simulink model "SystemQ"  (R2014b)
settings: Solver=ode23  StartTime=0.0  StopTime=inf  RelTol=10e-3
PreLoadFcn:
  | initSysQ;
  | runSysQ;
undefined symbols (not defined in the file): Controllers, CR, dim, fdesignblkfcn, G, gcbh, lib, serial, Tjoint, Tpid, X, Y, Z
libraries: sm_lib x62, nesl_utility x28, simulink x10, roblocks x5, instrumentlib x2, dspmathops x1, dspinverses x1, dspmtrx3 x1
(part 1 of 3)
settings Model: Creator=Flavio  LastModifiedBy=Edoardo

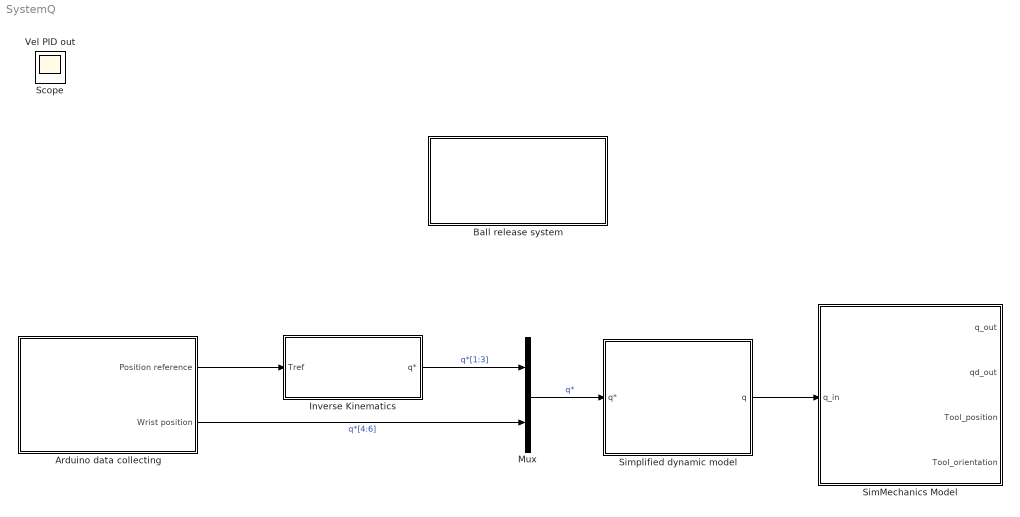
== system SystemQ ==
  Arduino data collecting : Subsystem
      mask Display:
      | image('Img/ardlogo.png',[0 0 0.75 1]);
      | port_label('output',1,'Pos. ref');
      | port_label('output',2,'Wrist joints');
  Ball release system : Subsystem
  Inverse Kinematics : Subsystem  mask{Jd=0.05, K=5}
      mask prompts: Jd "Jacobian damping"; K "Error gain"
  Mux : Mux  Inputs=2
  SimMechanics Model : Subsystem
      mask Display:
      | image('Img/simmech.png',[0.1 0.1 0.8 0.8]);
      | port_label('input',1,'q_in');
  Simplified dynamic model : Subsystem
      mask Display:
      | image('Img/dcmotor.jpg',[0.1 0.1 0.8 0.8]);
      | port_label('input',1,'q*');
      | port_label('output',1,'q');
  Scope : Scope
      settings: YMin=0  YMax=7  SaveName=ScopeData4
  Vel PID out : Scope
      settings: ShowLegends=on  YMin=-15  YMax=15  Decimation=10
  wires:
  Simplified dynamic model/1(q) -> SimMechanics Model/1("q_in ")
  Arduino data collecting/1(Position reference) -> Inverse Kinematics/1(Tref)
  Arduino data collecting/2(Wrist position) -> Mux/2  "q*[4:6]"
  Inverse Kinematics/1(q*) -> Mux/1  "q*[1:3]"
  Mux/1 -> Simplified dynamic model/1(q*)  "q*"

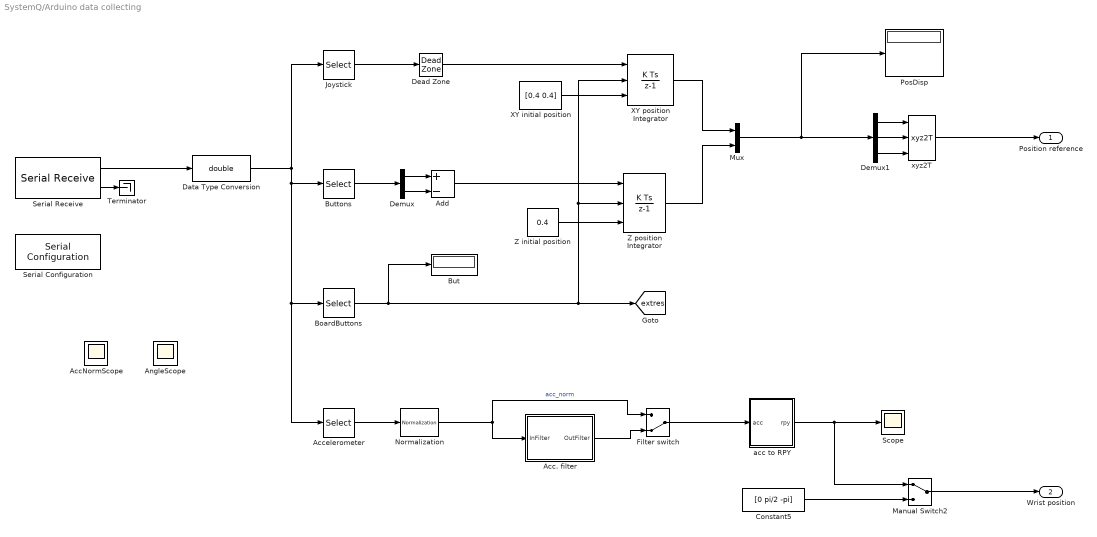
== system SystemQ/Arduino data collecting ==
  Acc. filter : Subsystem
  AccNormScope : Scope
      settings: Floating=on  ShowLegends=on  YMin=0  YMax=1  SaveName=ScopeData3
  Accelerometer : Selector  InputPortWidth=8  Indices=[5 6 7]
  Add : Sum  Inputs=+-
  AngleScope : Scope
      settings: Floating=on  ShowLegends=on  YMin=-0.2  YMax=1.6
  BoardButtons : Selector  InputPortWidth=8  Indices=8
  But : Display
  Buttons : Selector  InputPortWidth=8  Indices=[3 4]
  Constant5 : Constant  Value=[0 pi/2 -pi]
  Data Type Conversion : DataTypeConversion  OutDataTypeStr=double
  Dead Zone : DeadZone  LowerValue=-20  UpperValue=20  SaturateOnIntegerOverflow=on
  Demux : Demux  Outputs=2
  Demux1 : Demux  Outputs=3
  Filter switch : ManualSwitch  CurrentSetting=0
  Joystick : Selector  InputPortWidth=8  Indices=[1 2]
  Manual Switch2 : ManualSwitch
  Mux : Mux  Inputs=2
  Normalization : dspmathops/Normalization  NormType=2-norm  Bias=1e-10  NormOver=Each column  ColComp=on  Dimension=1  outputDataTypeStr=Inherit: Same as product output  outputLastDataTypeStr=Inherit: Same as product output  outputMin=[]  outputMax=[]  accumDataTypeStr=Inherit: Same as product output  accumLastDataTypeStr=Inherit: Same as product output  roundingMode=Floor  overflowMode=off
  PosDisp : Display
  Scope : Scope
      settings: SaveName=ScopeData2
  Serial Configuration : instrumentlib/Serial Configuration  Priority=-200000  ComPortMenu=<Please select a port...>  ComPort=COM5  ObjConstructor=serial('COM5');  BaudRate=115200  DataBits=8  Parity=none  StopBits=1  FlowControl=none  Timeout=10  ByteOrder=LittleEndian
  Serial Receive : instrumentlib/Serial Receive  ComPortMenu=<Please select a port...>  ComPort=COM5  ObjConstructor=serial('COM5');  Header=\a  Terminator=CR ('\r')  DataSize=8  DataType=int16  EnableBlockingMode=off  ActionDataUnavailable=Output last received value  CustomValue=0  SampleTime=0.1
  Terminator : Terminator
  XY initial position : Constant  Value=[0.4 0.4]
  XY position Integrator : DiscreteIntegrator  gainval=0.0001  ExternalReset=falling  InitialConditionSource=external  InitialCondition=[0.6181 0.4]  InitialConditionSetting=State (most efficient)  SampleTime=-1  UpperSaturationLimit=0.5  LowerSaturationLimit=-0.5
  Z initial position : Constant  Value=0.4
  Z position Integrator : DiscreteIntegrator  gainval=0.01  ExternalReset=falling  InitialConditionSource=external  InitialCondition=0.0875  InitialConditionSetting=State (most efficient)  SampleTime=-1  UpperSaturationLimit=0.6  LowerSaturationLimit=-0.6
  acc to RPY : Subsystem
  xyz2T : roblocks/Transform Conversion/xyz2T
  Position reference : Outport
  Wrist position : Outport  Port=2
  tag scope: extres=global
  wires:
  Demux1/1 -> xyz2T/1
  Add/1 -> Z position Integrator/1
  XY position Integrator/1 -> Mux/1
  Normalization/1 -> Filter switch/1, Acc. filter/1(InFilter)  "acc_norm"
  Data Type Conversion/1 -> BoardButtons/1, Accelerometer/1, Buttons/1, Joystick/1
  XY initial position/1 -> XY position Integrator/3
  Demux1/2 -> xyz2T/2
  Buttons/1 -> Demux/1
  Z position Integrator/1 -> Mux/2
  Joystick/1 -> Dead Zone/1
  Demux1/3 -> xyz2T/3
  Z initial position/1 -> Z position Integrator/3
  Mux/1 -> Demux1/1, PosDisp/1
  Dead Zone/1 -> XY position Integrator/1
  Filter switch/1 -> acc to RPY/1(acc)
  Acc. filter/1(OutFilter) -> Filter switch/2
  Demux/2 -> Add/2
  Demux/1 -> Add/1
  Accelerometer/1 -> Normalization/1
  Serial Receive/1 -> Data Type Conversion/1
  Serial Receive/2 -> Terminator/1
  xyz2T/1 -> Position reference/1
  Manual Switch2/1 -> Wrist position/1
  acc to RPY/1(rpy) -> Scope/1, Manual Switch2/1
  Constant5/1 -> Manual Switch2/2
  BoardButtons/1 -> But/1, XY position Integrator/2, Z position Integrator/2, [extres]

== system SystemQ/Ball release system ==
  BallChart : Stateflow chart  TreatAsAtomicUnit=on
  Memory error x : Memory  X0=1
  Memory error x1 : Memory  X0=1
  tag scope: Status=global
  wires:
  Memory error x/1 -> BallChart/1(error1)
  [ER1] -> Memory error x/1
  [ER2] -> Memory error x1/1
  Memory error x1/1 -> BallChart/2(error2)
  BallChart/1(status) -> [Status]

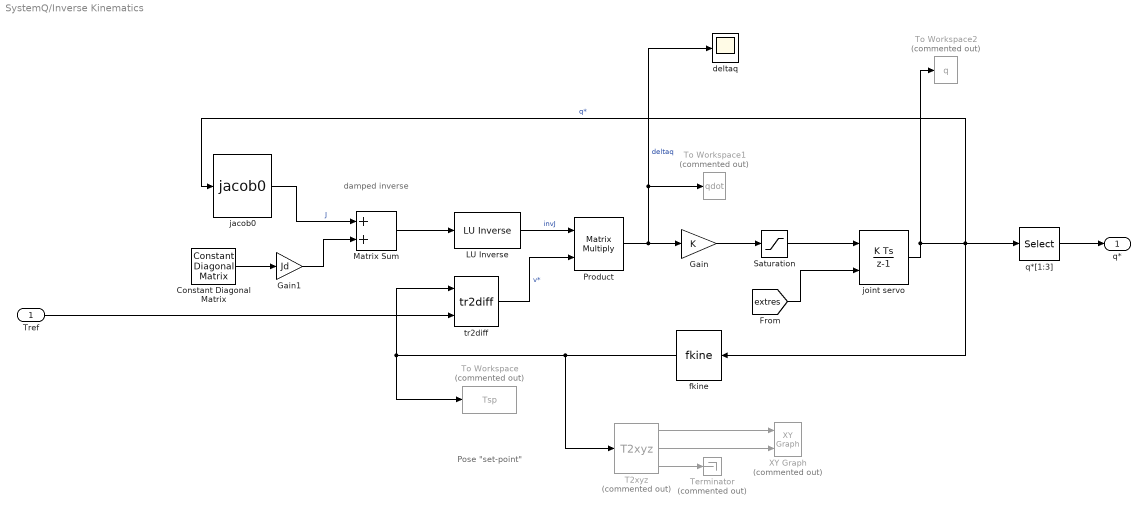
== system SystemQ/Inverse Kinematics ==
  note: Pose "set-point"
  note: damped inverse
  Tref : Inport
  " LU Inverse" : dspinverses/ LU Inverse
  Constant Diagonal Matrix : dspmtrx3/Constant Diagonal Matrix  q=ones(1,6)  frame=off  dataType=Inherit from 'Constant(s) along diagonal'  isSigned=on  wordLen=16  udDataType=sfix(16)  fracBitsMode=Best precision  numFracBits=15
  Gain : Gain  Gain=K  SaturateOnIntegerOverflow=on  OutDataTypeStr=Inherit: Same as input  ParamDataTypeStr=Inherit: Same as input
  Gain1 : Gain  Gain=Jd
  Matrix Sum : Sum
  Product : Product  Multiplication=Matrix(*)  SaturateOnIntegerOverflow=on  RndMeth=Zero  InputSameDT=on  OutDataTypeStr=Inherit: Same as first input
  Saturation : Saturate  UpperLimit=10  LowerLimit=-10
  T2xyz : roblocks/Transform Conversion/T2xyz  Commented=on
  Terminator : Terminator  Commented=on
  To Workspace : ToWorkspace  Commented=on  VariableName=Tsp  SampleTime=-1
  To Workspace1 : ToWorkspace  Commented=on  VariableName=qdot  SampleTime=-1
  To Workspace2 : ToWorkspace  Commented=on  VariableName=q  SampleTime=-1
  XY Graph : simulink/Sinks/XY Graph  Commented=on  xmin=-1  xmax=1  ymin=-1  ymax=1  st=-1
  deltaq : Scope
      settings: YMin=-2.5e-13  YMax=2.5e-13  SaveName=ScopeData7
  fkine : roblocks/Kinematics/fkine  robot=robot
  "jacob0 " : roblocks/Kinematics/jacob0   robot=robot
  joint servo : DiscreteIntegrator  ExternalReset=falling  InitialCondition=qn'  SampleTime=Tjoint  UpperSaturationLimit=pi  LowerSaturationLimit=-pi
  q*[1:3] : Selector  InputPortWidth=6  Indices=[1 2 3]
  tr2diff : roblocks/Kinematics/tr2diff  robot=robot
  q* : Outport
  wires:
  Constant Diagonal Matrix/1 -> Gain1/1
  Gain/1 -> Saturation/1
  " LU Inverse"/1 -> Product/1  "invJ"
  fkine/1 -> T2xyz/1, To Workspace/1, tr2diff/1
  Tref/1 -> tr2diff/2
  T2xyz/1 -> XY Graph/1
  Gain1/1 -> Matrix Sum/2
  "jacob0 "/1 -> Matrix Sum/1  "J"
  tr2diff/1 -> Product/2  "v*"
  T2xyz/2 -> XY Graph/2
  Matrix Sum/1 -> " LU Inverse"/1
  Product/1 -> deltaq/1, To Workspace1/1, Gain/1  "deltaq"
  T2xyz/3 -> Terminator/1
  joint servo/1 -> To Workspace2/1, fkine/1, "jacob0 "/1, q*[1:3]/1  "q*"
  [extres] -> joint servo/2
  Saturation/1 -> joint servo/1
  q*[1:3]/1 -> q*/1

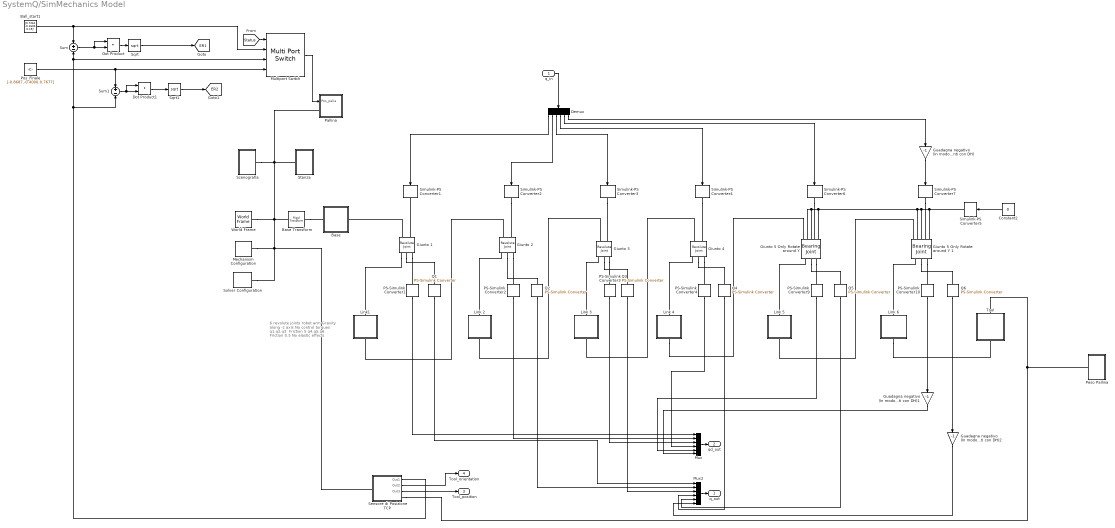
== system SystemQ/SimMechanics Model ==
  note: 6 revolute joints robot arm
      | Gravity along -z axis
      | No control torques
      | q1,q2,q3: Friction 5
      |  q4,q5,q6: Friction 0.5
      | No elastic effects
  "q_in " : Inport
  Ball_start1 : Constant  Value=[0.7261 -0.1604 0.15]'
  Base : Subsystem  mask(Double Pendulum Base){R=20, B_T=5, C_L=65, rp=5, clr=[0.5 0.5 0.5], Ro=dim.ro}
      mask prompts: R "Base radius (cm):"; B_T "Base thickeness (cm):"; C_L "Lunghezza cilindro (cm)"; rp "Peg radius (cm):"; clr "Base color:"; Ro "Densità (Kg/m^3):"
      mask help: Base body of the double pendulum mechanism.
  Base Transform : sm_lib/Frames and Transforms/Rigid Transform  TranslationMethod=None  TranslationLengthUnit=m  TranslationStandardAxis=+Z  TranslationStandardOffset=0  TranslationCartesianOffset=[0 0 0]  TranslationROffset=0  TranslationROffsetUnits=m  TranslationZOffset=0  TranslationZOffsetUnits=m  TranslationThetaOffset=0  TranslationThetaOffsetUnits=deg  RotationMethod=None  RotationAngleUnits=deg  RotationStandardAxis=+Z  RotationAngle=0  RotationArbitraryAxis=[0 0 1]  FollAlignAxisA=+Z  BaseAlignAxisA=-Y  FollAlignAxisB=+Y  BaseAlignAxisB=+X  RotationMatrix=[1 0 0; 0 1 0; 0 0 1]  BlockFunction=simmechanics.library.frames_transforms.rigid_transform
  Constant2 : Constant  Value=0
  Demux : Demux  Outputs=6
  Dot Product : DotProduct  InputSameDT=on  OutDataTypeStr=Inherit: Inherit via internal rule
  Dot Product1 : DotProduct  InputSameDT=on  OutDataTypeStr=Inherit: Inherit via internal rule
  Giunto 1 : sm_lib/Joints/Revolute Joint  SenseConstraintForce=off  SenseConstraintForceX=off  SenseConstraintForceY=off  SenseConstraintForceZ=off  SenseConstraintTorque=off  SenseConstraintTorqueX=off  SenseConstraintTorqueY=off  SenseConstraintTorqueZ=off  SenseTotalForce=off  SenseTotalForceX=off  SenseTotalForceY=off  SenseTotalForceZ=off  SenseTotalTorque=off  SenseTotalTorqueX=off  SenseTotalTorqueY=off  SenseTotalTorqueZ=off  CompositeWrenchDir=FollowerOnBase  CompositeWrenchFrame=BaseFrame  EquilibriumPosition=0  EquilibriumPositionUnits=rad  SpringStiffness=0  SpringStiffnessUnits=N*m/rad  DampingCoefficient=5  DampingCoefficientUnits=N*m/(rad/s)  TorqueActuationMode=ComputedTorque  MotionActuationMode=InputMotion  SensePosition=on  SenseVelocity=on  SenseAcceleration=off  SenseTorqueForce=off  PositionTargetValue=0  PositionTargetValueUnits=rad  PositionTargetSpecify=on  PositionTargetPriority=High  VelocityTargetValue=0  VelocityTargetValueUnits=rad/s  VelocityTargetSpecify=off  VelocityTargetPriority=Low  BlockFunction=simmechanics.library.joints.revolute_joint
  Giunto 2 : sm_lib/Joints/Revolute Joint  SenseConstraintForce=off  SenseConstraintForceX=off  SenseConstraintForceY=off  SenseConstraintForceZ=off  SenseConstraintTorque=off  SenseConstraintTorqueX=off  SenseConstraintTorqueY=off  SenseConstraintTorqueZ=off  SenseTotalForce=off  SenseTotalForceX=off  SenseTotalForceY=off  SenseTotalForceZ=off  SenseTotalTorque=off  SenseTotalTorqueX=off  SenseTotalTorqueY=off  SenseTotalTorqueZ=off  CompositeWrenchDir=FollowerOnBase  CompositeWrenchFrame=BaseFrame  EquilibriumPosition=0  EquilibriumPositionUnits=rad  SpringStiffness=0  SpringStiffnessUnits=N*m/rad  DampingCoefficient=5  DampingCoefficientUnits=N*m/(rad/s)  TorqueActuationMode=ComputedTorque  MotionActuationMode=InputMotion  SensePosition=on  SenseVelocity=on  SenseAcceleration=off  SenseTorqueForce=off  PositionTargetValue=pi/2  PositionTargetValueUnits=rad  PositionTargetSpecify=on  PositionTargetPriority=High  VelocityTargetValue=0  VelocityTargetValueUnits=rad/s  VelocityTargetSpecify=off  VelocityTargetPriority=Low  BlockFunction=simmechanics.library.joints.revolute_joint
  Giunto 3 : sm_lib/Joints/Revolute Joint  SenseConstraintForce=off  SenseConstraintForceX=off  SenseConstraintForceY=off  SenseConstraintForceZ=off  SenseConstraintTorque=off  SenseConstraintTorqueX=off  SenseConstraintTorqueY=off  SenseConstraintTorqueZ=off  SenseTotalForce=off  SenseTotalForceX=off  SenseTotalForceY=off  SenseTotalForceZ=off  SenseTotalTorque=off  SenseTotalTorqueX=off  SenseTotalTorqueY=off  SenseTotalTorqueZ=off  CompositeWrenchDir=FollowerOnBase  CompositeWrenchFrame=BaseFrame  EquilibriumPosition=pi/4  EquilibriumPositionUnits=rad  SpringStiffness=0  SpringStiffnessUnits=N*m/rad  DampingCoefficient=5  DampingCoefficientUnits=N*m/(rad/s)  TorqueActuationMode=ComputedTorque  MotionActuationMode=InputMotion  SensePosition=on  SenseVelocity=on  SenseAcceleration=off  SenseTorqueForce=off  PositionTargetValue=-(pi*5/6)  PositionTargetValueUnits=rad  PositionTargetSpecify=on  PositionTargetPriority=High  VelocityTargetValue=0  VelocityTargetValueUnits=rad/s  VelocityTargetSpecify=off  VelocityTargetPriority=Low  BlockFunction=simmechanics.library.joints.revolute_joint
  Giunto 4 : sm_lib/Joints/Revolute Joint  SenseConstraintForce=off  SenseConstraintForceX=off  SenseConstraintForceY=off  SenseConstraintForceZ=off  SenseConstraintTorque=off  SenseConstraintTorqueX=off  SenseConstraintTorqueY=off  SenseConstraintTorqueZ=off  SenseTotalForce=off  SenseTotalForceX=off  SenseTotalForceY=off  SenseTotalForceZ=off  SenseTotalTorque=off  SenseTotalTorqueX=off  SenseTotalTorqueY=off  SenseTotalTorqueZ=off  CompositeWrenchDir=FollowerOnBase  CompositeWrenchFrame=BaseFrame  EquilibriumPosition=0  EquilibriumPositionUnits=rad  SpringStiffness=0  SpringStiffnessUnits=N*m/rad  DampingCoefficient=0.5  DampingCoefficientUnits=N*m/(rad/s)  TorqueActuationMode=ComputedTorque  MotionActuationMode=InputMotion  SensePosition=on  SenseVelocity=on  SenseAcceleration=off  SenseTorqueForce=off  PositionTargetValue=0  PositionTargetValueUnits=rad  PositionTargetSpecify=on  PositionTargetPriority=High  VelocityTargetValue=0  VelocityTargetValueUnits=rad/s  VelocityTargetSpecify=off  VelocityTargetPriority=Low  BlockFunction=simmechanics.library.joints.revolute_joint
  "Giunto 5 Only Rotate around Y " : sm_lib/Joints/Bearing Joint  SenseConstraintForce=off  SenseConstraintForceX=off  SenseConstraintForceY=off  SenseConstraintForceZ=off  SenseConstraintTorque=off  SenseConstraintTorqueX=off  SenseConstraintTorqueY=off  SenseConstraintTorqueZ=off  SenseTotalForce=off  SenseTotalForceX=off  SenseTotalForceY=off  SenseTotalForceZ=off  SenseTotalTorque=off  SenseTotalTorqueX=off  SenseTotalTorqueY=off  SenseTotalTorqueZ=off  CompositeWrenchDir=FollowerOnBase  CompositeWrenchFrame=BaseFrame  PzEquilibriumPosition=0  PzEquilibriumPositionUnits=m  PzSpringStiffness=0  PzSpringStiffnessUnits=N/m  PzDampingCoefficient=0  PzDampingCoefficientUnits=N/(m/s)  PzTorqueActuationMode=ComputedTorque  PzMotionActuationMode=InputMotion  PzSensePosition=off  PzSenseVelocity=off  PzSenseAcceleration=off  PzSenseTorqueForce=off  PzPositionTargetValue=0  PzPositionTargetValueUnits=m  PzPositionTargetSpecify=on  PzPositionTargetPriority=High  PzVelocityTargetValue=0  PzVelocityTargetValueUnits=m/s  PzVelocityTargetSpecify=off  PzVelocityTargetPriority=High  RxEquilibriumPosition=0  RxEquilibriumPositionUnits=deg  RxSpringStiffness=0  RxSpringStiffnessUnits=N*m/deg  RxDampingCoefficient=0  RxDampingCoefficientUnits=N*m/(deg/s)  RxTorqueActuationMode=ComputedTorque  RxMotionActuationMode=InputMotion  RxSensePosition=off  RxSenseVelocity=off  RxSenseAcceleration=off  RxSenseTorqueForce=off  RxPositionTargetValue=0  RxPositionTargetValueUnits=rad  RxPositionTargetSpecify=on  RxPositionTargetPriority=High  RxVelocityTargetValue=0  RxVelocityTargetValueUnits=deg/s  RxVelocityTargetSpecify=off  RxVelocityTargetPriority=High  RyEquilibriumPosition=0  RyEquilibriumPositionUnits=deg  RySpringStiffness=0  RySpringStiffnessUnits=N*m/deg  RyDampingCoefficient=0.5  RyDampingCoefficientUnits=N*m/(rad/s)  RyTorqueActuationMode=ComputedTorque  RyMotionActuationMode=InputMotion  RySensePosition=on  RySenseVelocity=on  RySenseAcceleration=off  RySenseTorqueForce=off  RyPositionTargetValue=pi/6  RyPositionTargetValueUnits=rad  RyPositionTargetSpecify=on  RyPositionTargetPriority=High  RyVelocityTargetValue=0  RyVelocityTargetValueUnits=deg/s  RyVelocityTargetSpecify=off  RyVelocityTargetPriority=High  RzEquilibriumPosition=0  RzEquilibriumPositionUnits=deg  RzSpringStiffness=0  RzSpringStiffnessUnits=N*m/deg  RzDampingCoefficient=0  RzDampingCoefficientUnits=N*m/(deg/s)  RzTorqueActuationMode=ComputedTorque  RzMotionActuationMode=InputMotion  RzSensePosition=off  RzSenseVelocity=off  RzSenseAcceleration=off  RzSenseTorqueForce=off  RzPositionTargetValue=0  RzPositionTargetValueUnits=rad  RzPositionTargetSpecify=on  RzPositionTargetPriority=High  RzVelocityTargetValue=0  RzVelocityTargetValueUnits=deg/s  RzVelocityTargetSpecify=off  RzVelocityTargetPriority=High  BlockFunction=simmechanics.library.joints.bearing_joint
  Giunto 5 Only Rotate around Y 1 : sm_lib/Joints/Bearing Joint  SenseConstraintForce=off  SenseConstraintForceX=off  SenseConstraintForceY=off  SenseConstraintForceZ=off  SenseConstraintTorque=off  SenseConstraintTorqueX=off  SenseConstraintTorqueY=off  SenseConstraintTorqueZ=off  SenseTotalForce=off  SenseTotalForceX=off  SenseTotalForceY=off  SenseTotalForceZ=off  SenseTotalTorque=off  SenseTotalTorqueX=off  SenseTotalTorqueY=off  SenseTotalTorqueZ=off  CompositeWrenchDir=FollowerOnBase  CompositeWrenchFrame=BaseFrame  PzEquilibriumPosition=0  PzEquilibriumPositionUnits=m  PzSpringStiffness=0  PzSpringStiffnessUnits=N/m  PzDampingCoefficient=0  PzDampingCoefficientUnits=N/(m/s)  PzTorqueActuationMode=ComputedTorque  PzMotionActuationMode=InputMotion  PzSensePosition=off  PzSenseVelocity=off  PzSenseAcceleration=off  PzSenseTorqueForce=off  PzPositionTargetValue=0  PzPositionTargetValueUnits=m  PzPositionTargetSpecify=on  PzPositionTargetPriority=High  PzVelocityTargetValue=0  PzVelocityTargetValueUnits=m/s  PzVelocityTargetSpecify=off  PzVelocityTargetPriority=High  RxEquilibriumPosition=0  RxEquilibriumPositionUnits=deg  RxSpringStiffness=0  RxSpringStiffnessUnits=N*m/deg  RxDampingCoefficient=0  RxDampingCoefficientUnits=N*m/(deg/s)  RxTorqueActuationMode=ComputedTorque  RxMotionActuationMode=InputMotion  RxSensePosition=off  RxSenseVelocity=off  RxSenseAcceleration=off  RxSenseTorqueForce=off  RxPositionTargetValue=0  RxPositionTargetValueUnits=rad  RxPositionTargetSpecify=on  RxPositionTargetPriority=High  RxVelocityTargetValue=0  RxVelocityTargetValueUnits=deg/s  RxVelocityTargetSpecify=off  RxVelocityTargetPriority=High  RyEquilibriumPosition=0  RyEquilibriumPositionUnits=deg  RySpringStiffness=0  RySpringStiffnessUnits=N*m/deg  RyDampingCoefficient=0.5  RyDampingCoefficientUnits=N*m/(rad/s)  RyTorqueActuationMode=ComputedTorque  RyMotionActuationMode=InputMotion  RySensePosition=on  RySenseVelocity=on  RySenseAcceleration=off  RySenseTorqueForce=off  RyPositionTargetValue=0  RyPositionTargetValueUnits=rad  RyPositionTargetSpecify=on  RyPositionTargetPriority=High  RyVelocityTargetValue=0  RyVelocityTargetValueUnits=deg/s  RyVelocityTargetSpecify=off  RyVelocityTargetPriority=High  RzEquilibriumPosition=0  RzEquilibriumPositionUnits=deg  RzSpringStiffness=0  RzSpringStiffnessUnits=N*m/deg  RzDampingCoefficient=0  RzDampingCoefficientUnits=N*m/(deg/s)  RzTorqueActuationMode=ComputedTorque  RzMotionActuationMode=InputMotion  RzSensePosition=off  RzSenseVelocity=off  RzSenseAcceleration=off  RzSenseTorqueForce=off  RzPositionTargetValue=0  RzPositionTargetValueUnits=rad  RzPositionTargetSpecify=on  RzPositionTargetPriority=High  RzVelocityTargetValue=0  RzVelocityTargetValueUnits=deg/s  RzVelocityTargetSpecify=off  RzVelocityTargetPriority=High  BlockFunction=simmechanics.library.joints.bearing_joint
  Guadagna negativo (In modo da avere il verso di rotazione coerenti con DH) : Gain  Gain=-1
  Guadagna negativo (In modo da avere il verso di rotazione coerenti con DH)1 : Gain  Gain=-1
  Guadagna negativo (In modo da avere il verso di rotazione coerenti con DH)2 : Gain  Gain=-1
  Link 2 : Subsystem  mask{C_L=dim.L2*100, C_R=5, Ro=dim.ro}
      mask prompts: C_L "Lunghezza Braccio (cm):"; C_R "Lunghezza Cardine (cm):"; Ro "Densità (Kg/m^3):"
  Link 3 : Subsystem  mask{C_2_L=dim.L3*100, C_L=15, Ro=dim.ro}
      mask prompts: C_2_L "Lunghezza Braccio (cm):"; C_L "Lunghezza Cardine (cm):"; Ro "Densità (Kg/m^3):"
  Link 4 : Subsystem  mask{Ro=dim.ro}
      mask prompts: Ro "Densità (Kg/m^3):"
  Link 5 : Subsystem  mask{Ro=dim.ro}
      mask prompts: Ro "Densità (Kg/m^3):"
  Link 6 : Subsystem  mask{Ro=dim.ro}
      mask prompts: Ro "Densità (Kg/m^3):"
  Link1 : Subsystem  mask{C_L=dim.L1*100, C_R=5, Ro=dim.ro}
      mask prompts: C_L "Lunghezza Braccio (cm):"; C_R "Lunghezza Cardine (cm):"; Ro "Densità (Kg/m^3):"
  Mechanism Configuration : sm_lib/Utilities/Mechanism Configuration  UniformGravity=Constant  GravityVector=[0 0 -G]  GravityUnits=m/s^2  LinearizationDelta=0.001  BlockFunction=simmechanics.library.utilities.mechanism_configuration
  Multiport Switch : MultiPortSwitch  DataPortOrder=Zero-based contiguous
  Mux : Mux  Inputs=6
  Mux2 : Mux  Inputs=6
  PS-Simulink Converter{1..4,9..10} (6 alike) : nesl_utility/PS-Simulink Converter  PhysicalDomain=network_engine_domain  SubClassName=ps_output  LeftPortType=input  RightPortType=output  PseudoPeriodic=off  Frequencies=[]  Unit=rad/s  AffineConversion=off
  Pallina : Subsystem
  Peso Pallina : Subsystem
  Pos_Finale : Constant  Value=[-0.8687,-0.4000,0.7677]
  Q{1..6} (6 alike) : nesl_utility/PS-Simulink Converter  PhysicalDomain=network_engine_domain  SubClassName=ps_output  LeftPortType=input  RightPortType=output  PseudoPeriodic=off  Frequencies=[]  Unit=rad  AffineConversion=off
  Scenografia : Subsystem
  Sensore di Posizione TCP : Subsystem
  Simulink-PS Converter{1..4,6..7} (6 alike) : nesl_utility/Simulink-PS Converter  PhysicalDomain=network_engine_domain  SubClassName=ps_input  LeftPortType=input  RightPortType=output  PseudoPeriodic=off  Frequencies=[]  NoiseDistribution=none  NoiseParameters=[]  Unit=rad  AffineConversion=off  InputFiltering=on  SimscapeFilterOrder=2  InputFilterTimeConstant=0.001  UdotUserProvided=1
  Simulink-PS Converter5 : nesl_utility/Simulink-PS Converter  PhysicalDomain=network_engine_domain  SubClassName=ps_input  LeftPortType=input  RightPortType=output  PseudoPeriodic=off  Frequencies=[]  NoiseDistribution=none  NoiseParameters=[]  Unit=1  AffineConversion=off  InputFiltering=off  SimscapeFilterOrder=1  InputFilterTimeConstant=0.001  UdotUserProvided=1
  Solver Configuration : nesl_utility/Solver Configuration  PhysicalDomain=network_engine_domain  SubClassName=solver  LeftPortType=input  RightPortType=generic  Accelerate=off  Tones=[]  Harmonics=[]  SimulateNoise=off  Profile=off  UseLocalSampling=off  EnableSwitchedLinearOptims=on  FrequencyDomain=off  UseCCode=off  RelTol=0.001  AbsTol=1e-06  MinStep=1e-09  ToWorkspace=off  DoDC=off  ResidualTolerance=1e-9  UseLocalSolver=on  LocalSolverChoice=NE_BACKWARD_EULER_ADVANCER  LocalSolverSampleTime=0.001  DoFixedCost=on  MaxNonlinIter=3  MaxModeIter=2  LinearAlgebra=Full  DelaysMemoryBudget=1024  AutomaticFiltering=on  FilteringTimeConstant=0.001
  Sqrt : Sqrt  SaturateOnIntegerOverflow=on
  Sqrt1 : Sqrt  SaturateOnIntegerOverflow=on
  Stanza : Subsystem
  Sum : Sum  Inputs=+-
  Sum1 : Sum  Inputs=+-
  Tool : Subsystem  mask{Ro=0}
      mask prompts: Ro "Densità (Kg/m^3):"
  World Frame : sm_lib/Frames and Transforms/World Frame  BlockFunction=simmechanics.library.frames_transforms.world_frame
  q_out : Outport
  qd_out : Outport  Port=2
  Tool_position : Outport  Port=3
  Tool_orientation : Outport  Port=4
  tag scope: ER1=global, ER2=global
  wires:
  Q6/1 -> Guadagna negativo (In modo da avere il verso di rotazione coerenti con DH)2/1
  Q5/1 -> Mux2/5
  Q4/1 -> Mux2/4
  Q3/1 -> Mux2/3
  Q2/1 -> Mux2/2
  Q1/1 -> Mux2/1
  Mux2/1 -> q_out/1
  Guadagna negativo (In modo da avere il verso di rotazione coerenti con DH)1/1 -> Mux/6
  Guadagna negativo (In modo da avere il verso di rotazione coerenti con DH)/1 -> Simulink-PS Converter7/1
  Demux/6 -> Guadagna negativo (In modo da avere il verso di rotazione coerenti con DH)/1
  "q_in "/1 -> Demux/1
  Demux/5 -> Simulink-PS Converter6/1
  Demux/4 -> Simulink-PS Converter4/1
  Demux/3 -> Simulink-PS Converter3/1
  Demux/2 -> Simulink-PS Converter2/1
  Demux/1 -> Simulink-PS Converter1/1
  Mux/1 -> qd_out/1
  PS-Simulink Converter10/1 -> Guadagna negativo (In modo da avere il verso di rotazione coerenti con DH)1/1
  PS-Simulink Converter9/1 -> Mux/5
  PS-Simulink Converter4/1 -> Mux/4
  PS-Simulink Converter3/1 -> Mux/3
  PS-Simulink Converter2/1 -> Mux/2
  PS-Simulink Converter1/1 -> Mux/1
  Constant2/1 -> Simulink-PS Converter5/1
  Guadagna negativo (In modo da avere il verso di rotazione coerenti con DH)2/1 -> Mux2/6
  Sensore di Posizione TCP/2(Out2) -> Tool_orientation/1
  Sensore di Posizione TCP/3(Out3) -> Tool_position/1
  Dot Product/1 -> Sqrt/1
  Sum/1 -> Dot Product/1, Dot Product/2
  Sensore di Posizione TCP/1(Out1) -> Sum1/2, Multiport Switch/3, Sum/2
  Ball_start1/1 -> Sum/1, Multiport Switch/2
  Pos_Finale/1 -> Sum1/1, Multiport Switch/4
  Dot Product1/1 -> Sqrt1/1
  Sum1/1 -> Dot Product1/1, Dot Product1/2
  Sqrt/1 -> [ER1]
  Sqrt1/1 -> [ER2]
  Multiport Switch/1 -> Pallina/1(Pos_palla)
  [Status] -> Multiport Switch/1
  connections:
  Link 6/RConn1 -- Tool/RConn1
  Giunto 5 Only Rotate around Y 1/RConn3 -- PS-Simulink Converter10/LConn1
  Giunto 5 Only Rotate around Y 1/RConn2 -- Q6/LConn1
  "Giunto 5 Only Rotate around Y "/RConn3 -- PS-Simulink Converter9/LConn1
  "Giunto 5 Only Rotate around Y "/RConn2 -- Q5/LConn1
  Giunto 4/RConn3 -- PS-Simulink Converter4/LConn1
  Giunto 4/RConn2 -- Q4/LConn1
  Giunto 3/RConn3 -- PS-Simulink Converter3/LConn1
  Giunto 3/RConn2 -- Q3/LConn1
  Giunto 2/RConn2 -- Q2/LConn1
  Giunto 2/RConn3 -- PS-Simulink Converter2/LConn1
  Giunto 1/RConn2 -- Q1/LConn1
  Giunto 1/RConn3 -- PS-Simulink Converter1/LConn1
  Simulink-PS Converter7/RConn1 -- Giunto 5 Only Rotate around Y 1/LConn4
  Giunto 5 Only Rotate around Y 1/RConn1 -- Link 6/LConn1
  Simulink-PS Converter6/RConn1 -- "Giunto 5 Only Rotate around Y "/LConn4
  Simulink-PS Converter4/RConn1 -- Giunto 4/LConn2
  Simulink-PS Converter3/RConn1 -- Giunto 3/LConn2
  Simulink-PS Converter2/RConn1 -- Giunto 2/LConn2
  Simulink-PS Converter5/RConn1 -- Giunto 5 Only Rotate around Y 1/LConn5 -- Giunto 5 Only Rotate around Y 1/LConn3 -- Giunto 5 Only Rotate around Y 1/LConn2 -- "Giunto 5 Only Rotate around Y "/LConn3 -- "Giunto 5 Only Rotate around Y "/LConn2 -- "Giunto 5 Only Rotate around Y "/LConn5
  Giunto 5 Only Rotate around Y 1/LConn1 -- Link 5/RConn1
  Link 4/RConn1 -- "Giunto 5 Only Rotate around Y "/LConn1
  Giunto 4/LConn1 -- Link 3/RConn1
  Giunto 1/LConn1 -- Base/RConn1
  Giunto 3/RConn1 -- Link 3/LConn1
  Giunto 3/LConn1 -- Link 2/RConn1
  Base Transform/RConn1 -- Base/LConn1
  Giunto 2/LConn1 -- Link1/RConn1
  Giunto 2/RConn1 -- Link 2/LConn1
  Giunto 4/RConn1 -- Link 4/LConn1
  "Giunto 5 Only Rotate around Y "/RConn1 -- Link 5/LConn1
  Giunto 1/LConn2 -- Simulink-PS Converter1/RConn1
  Giunto 1/RConn1 -- Link1/LConn1
  Scenografia/RConn1 -- Sensore di Posizione TCP/LConn1 -- Mechanism Configuration/RConn1 -- Solver Configuration/RConn1 -- World Frame/RConn1 -- Base Transform/LConn1 -- Pallina/LConn1 -- Stanza/RConn1
  Sensore di Posizione TCP/RConn1 -- Peso Pallina/LConn1 -- Tool/LConn1

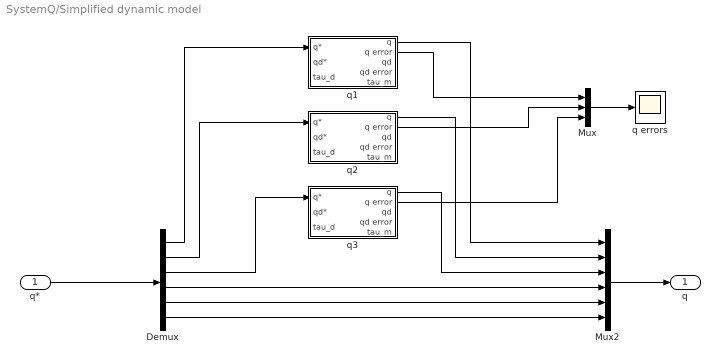
== system SystemQ/Simplified dynamic model ==
  q* : Inport
  Demux : Demux  Outputs=6
  Mux : Mux  Inputs=3
  Mux2 : Mux  Inputs=6
  q errors : Scope
      settings: YMin=-15  YMax=10  SaveName=ScopeData5
  q1 : Subsystem  AncestorBlock=lib/Controllers  mask{Kt=0.228, tau_max=0.9, Jm=200e-6, Jl=2, G=100, B=817e-6, omega_max=165, Kp_v=1, Ki_v=1, Kd_v=0, Kp_p=20, Ki_p=0, Kd_p=0, Kff_p=0, Ts=Tpid}
      mask prompts: Kt "Motor torque constant (Kt) [Nm/A]"; tau_max "Max torque (tau_max) [Nm]"; Jm "Motor shaft inertia (Jm) [kg*m^2]"; Jl "Load inertia (Jl) [kg*m^2]"; G "Gearbox transformation ratio (G)"; B "Motor viscous friction (B) [Nm*s/rad]"; omega_max "Max speed (omega_max) [rad/s]"; Kp_v "Proportional gain (Kp)"; Ki_v "Integral gain (Ki)"; Kd_v "Derivative gain (Kd)"; Kp_p "Proportional gain (Kp)"; Ki_p "Integral gain (Ki)"; Kd_p "Derivative gain (Kd)"; Kff_p "Feedforward gain (Kff)"; Ts "Sample time (Ts)"
      mask DialogControl Container7 Prompt: Velocity loop
      mask DialogControl Container9 Prompt: Position loop
  q2 : Subsystem  AncestorBlock=lib/Controllers  mask{Kt=0.228, tau_max=0.9, Jm=200e-6, Jl=1, G=100, B=817e-6, omega_max=165, Kp_v=1, Ki_v=5, Kd_v=0, Kp_p=20, Ki_p=0, Kd_p=0, Kff_p=0, Ts=Tpid}
      mask prompts: Kt "Motor torque constant (Kt) [Nm/A]"; tau_max "Max torque (tau_max) [Nm]"; Jm "Motor shaft inertia (Jm) [kg*m^2]"; Jl "Load inertia (Jl) [kg*m^2]"; G "Gearbox transformation ratio (G)"; B "Motor viscous friction (B) [Nm*s/rad]"; omega_max "Max speed (omega_max) [rad/s]"; Kp_v "Proportional gain (Kp)"; Ki_v "Integral gain (Ki)"; Kd_v "Derivative gain (Kd)"; Kp_p "Proportional gain (Kp)"; Ki_p "Integral gain (Ki)"; Kd_p "Derivative gain (Kd)"; Kff_p "Feedforward gain (Kff)"; Ts "Sample time (Ts)"
      mask DialogControl Container7 Prompt: Velocity loop
      mask DialogControl Container9 Prompt: Position loop
  q3 : Subsystem  AncestorBlock=lib/Controllers  mask{Kt=0.228, tau_max=0.9, Jm=200e-6, Jl=0.5, G=100, B=817e-6, omega_max=165, Kp_v=1, Ki_v=5, Kd_v=0, Kp_p=20, Ki_p=0, Kd_p=0, Kff_p=0, Ts=Tpid}
      mask prompts: Kt "Motor torque constant (Kt) [Nm/A]"; tau_max "Max torque (tau_max) [Nm]"; Jm "Motor shaft inertia (Jm) [kg*m^2]"; Jl "Load inertia (Jl) [kg*m^2]"; G "Gearbox transformation ratio (G)"; B "Motor viscous friction (B) [Nm*s/rad]"; omega_max "Max speed (omega_max) [rad/s]"; Kp_v "Proportional gain (Kp)"; Ki_v "Integral gain (Ki)"; Kd_v "Derivative gain (Kd)"; Kp_p "Proportional gain (Kp)"; Ki_p "Integral gain (Ki)"; Kd_p "Derivative gain (Kd)"; Kff_p "Feedforward gain (Kff)"; Ts "Sample time (Ts)"
      mask DialogControl Container7 Prompt: Velocity loop
      mask DialogControl Container9 Prompt: Position loop
  q : Outport
  wires:
  Demux/4 -> Mux2/4
  q1/1(q) -> Mux2/1
  Demux/1 -> q1/1(q*)
  Mux2/1 -> q/1
  Demux/2 -> q2/1(q*)
  q3/1(q) -> Mux2/3
  q2/1(q) -> Mux2/2
  Demux/5 -> Mux2/5
  Demux/6 -> Mux2/6
  Demux/3 -> q3/1(q*)
  q2/2(q error) -> Mux/2
  q3/2(q error) -> Mux/3
  Mux/1 -> q errors/1
  q1/2(q error) -> Mux/1
  q*/1 -> Demux/1

== system SystemQ/Arduino data collecting/Acc. filter ==
  InFilter : Inport
  Demux : Demux  Outputs=3
  Lowpass Filter : Subsystem  DialogController=fdesignblkfcn  InitFcn=fdesignblkfcn(gcbh, {'InitFcn'});  mask(Lowpass Filter){}
      mask help: Design a lowpass filter
      settings: CopyFcn=fdesignblkfcn(gcbh, {'CopyFcn'});
      mask Help: helpview(mapfilelocation('dsp'), 'dsplowpassfilter');
      mask Display: disp('Lowpass')
  Lowpass Filter1 : Subsystem  DialogController=fdesignblkfcn  InitFcn=fdesignblkfcn(gcbh, {'InitFcn'});  mask(Lowpass Filter){}
      mask help: Design a lowpass filter
      settings: CopyFcn=fdesignblkfcn(gcbh, {'CopyFcn'});
      mask Help: helpview(mapfilelocation('dsp'), 'dsplowpassfilter');
      mask Display: disp('Lowpass')
  Lowpass Filter2 : Subsystem  DialogController=fdesignblkfcn  InitFcn=fdesignblkfcn(gcbh, {'InitFcn'});  mask(Lowpass Filter){}
      mask help: Design a lowpass filter
      settings: CopyFcn=fdesignblkfcn(gcbh, {'CopyFcn'});
      mask Help: helpview(mapfilelocation('dsp'), 'dsplowpassfilter');
      mask Display: disp('Lowpass')
  Mux : Mux  Inputs=3
  OutFilter : Outport
  wires:
  InFilter/1 -> Demux/1
  Demux/1 -> Lowpass Filter/1(In)
  Mux/1 -> OutFilter/1
  Lowpass Filter/1(Out) -> Mux/1  "acc_xf"
  Demux/2 -> Lowpass Filter1/1(In)
  Demux/3 -> Lowpass Filter2/1(In)
  Lowpass Filter1/1(Out) -> Mux/2
  Lowpass Filter2/1(Out) -> Mux/3

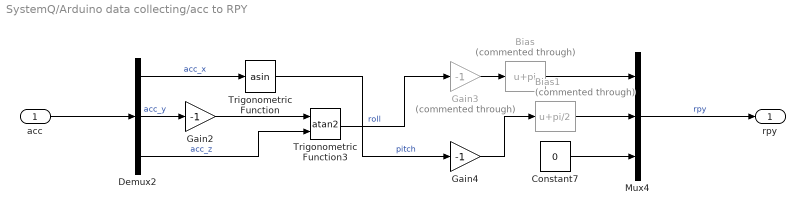
== system SystemQ/Arduino data collecting/acc to RPY ==
  acc : Inport
  Bias : Bias  Commented=through  Bias=pi
  Bias1 : Bias  Commented=through  Bias=pi/2
  Constant7 : Constant  Value=0
  Demux2 : Demux  Outputs=3
  Gain2 : Gain  Gain=-1
  Gain3 : Gain  Commented=through  Gain=-1
  Gain4 : Gain  Gain=-1
  Mux4 : Mux  Inputs=3
  Trigonometric Function : Trigonometry  Operator=asin  OutputSignalType=real
  Trigonometric Function3 : Trigonometry  Operator=atan2  OutputSignalType=real
  rpy : Outport
  wires:
  Mux4/1 -> rpy/1  "rpy"
  Constant7/1 -> Mux4/3
  Gain4/1 -> Bias1/1
  Gain3/1 -> Bias/1
  Bias/1 -> Mux4/1
  Demux2/2 -> Gain2/1  "acc_y"
  Demux2/1 -> Trigonometric Function/1  "acc_x"
  Demux2/3 -> Trigonometric Function3/2  "acc_z"
  Gain2/1 -> Trigonometric Function3/1
  Trigonometric Function/1 -> Gain4/1  "pitch"
  acc/1 -> Demux2/1
  Trigonometric Function3/1 -> Gain3/1  "roll"
  Bias1/1 -> Mux4/2

== system SystemQ/SimMechanics Model/Base ==
  Base : sm_lib/Body Elements/Solid  InertiaType=CalculateFromGeometry  Mass=1  MassUnits=kg  CenterOfMass=[0 0 0]  CenterOfMassUnits=m  MomentsOfInertia=[1 1 1]  MomentsOfInertiaUnits=kg*m^2  ProductsOfInertia=[0 0 0]  ProductsOfInertiaUnits=kg*m^2  DensityBased=on  Density=Ro  DensityUnits=kg/(m^3)  GraphicType=FromGeometry  MarkerShape=Sphere  MarkerSize=1  MarkerSizeUnits=m  GraphicVisPropType=SimpleVisualProperties  GraphicDiffuseColor=clr  GraphicSpecularColor=[0.2 0.2 0.2]  GraphicAmbientColor=[0.5 0.5 0.5]  GraphicEmissiveColor=[0.1 0.1 0.1]  GraphicShininess=24.0  GraphicOpacity=1  GeometryShape=RegularExtrusion  RectangleSize=[1 1]  RectangleSizeUnits=m  BrickDimensions=[1 1 1]  BrickDimensionUnits=m  CylinderRadius=1  CylinderRadiusUnits=m  CylinderLength=1  CylinderLengthUnits=m  SphereRadius=1  SphereRadiusUnits=m  EllipsoidRadii=[1 1 1]  EllipsoidRadiiUnits=m  ExtrusionCrossSection=[1 1; -1 1; -1 -1; 1 -1]  ExtrusionCrossSectionUnits=m  ExtrusionLength=B_T  ExtrusionLengthUnits=cm  PolygonNumSides=6  PolygonOuterRadius=R  PolygonOuterRadiusUnits=cm  ExtGeomFileType=STL  ExtGeomFileUnits=m  RevolutionCrossSection=[1 1; 1 -1; 2 -1; 2 1]  RevolutionCrossSectionUnits=m  RevolutionExtent=Full  RevolutionAngle=180  RevolutionAngleUnits=deg  BlockFunction=simmechanics.library.body_elements.solid
  Peg : sm_lib/Body Elements/Solid  InertiaType=CalculateFromGeometry  Mass=1  MassUnits=kg  CenterOfMass=[0 0 0]  CenterOfMassUnits=m  MomentsOfInertia=[1 1 1]  MomentsOfInertiaUnits=kg*m^2  ProductsOfInertia=[0 0 0]  ProductsOfInertiaUnits=kg*m^2  DensityBased=on  Density=Ro  DensityUnits=kg/(m^3)  GraphicType=FromGeometry  MarkerShape=Sphere  MarkerSize=1  MarkerSizeUnits=m  GraphicVisPropType=SimpleVisualProperties  GraphicDiffuseColor=clr  GraphicSpecularColor=[0.2 0.2 0.2]  GraphicAmbientColor=[0.5 0.5 0.5]  GraphicEmissiveColor=[0.1 0.1 0.1]  GraphicShininess=24.0  GraphicOpacity=1  GeometryShape=Cylinder  RectangleSize=[1 1]  RectangleSizeUnits=m  BrickDimensions=[1 1 1]  BrickDimensionUnits=m  CylinderRadius=rp  CylinderRadiusUnits=cm  CylinderLength=C_L  CylinderLengthUnits=cm  SphereRadius=1  SphereRadiusUnits=m  EllipsoidRadii=[1 1 1]  EllipsoidRadiiUnits=m  ExtrusionCrossSection=[1 1; -1 1; -1 -1; 1 -1]  ExtrusionCrossSectionUnits=m  ExtrusionLength=1  ExtrusionLengthUnits=m  PolygonNumSides=1  PolygonOuterRadius=1  PolygonOuterRadiusUnits=m  ExtGeomFileType=STL  ExtGeomFileUnits=m  RevolutionCrossSection=[1 1; 1 -1; 2 -1; 2 1]  RevolutionCrossSectionUnits=m  RevolutionExtent=Full  RevolutionAngle=180  RevolutionAngleUnits=deg  BlockFunction=simmechanics.library.body_elements.solid
  Peg center transform1 : sm_lib/Frames and Transforms/Rigid Transform  TranslationMethod=StandardAxis  TranslationLengthUnit=cm  TranslationStandardAxis=+Z  TranslationStandardOffset=B_T/2  TranslationCartesianOffset=[0 0 0]  TranslationROffset=0  TranslationROffsetUnits=m  TranslationZOffset=0  TranslationZOffsetUnits=m  TranslationThetaOffset=0  TranslationThetaOffsetUnits=deg  RotationMethod=None  RotationAngleUnits=deg  RotationStandardAxis=+Z  RotationAngle=0  RotationArbitraryAxis=[0 0 1]  FollAlignAxisA=+X  BaseAlignAxisA=+Y  FollAlignAxisB=+Y  BaseAlignAxisB=+Z  RotationMatrix=[1 0 0; 0 1 0; 0 0 1]  BlockFunction=simmechanics.library.frames_transforms.rigid_transform
  Peg center transform2 : sm_lib/Frames and Transforms/Rigid Transform  TranslationMethod=StandardAxis  TranslationLengthUnit=cm  TranslationStandardAxis=+Z  TranslationStandardOffset=C_L/2+B_T/2  TranslationCartesianOffset=[0 0 0]  TranslationROffset=0  TranslationROffsetUnits=m  TranslationZOffset=0  TranslationZOffsetUnits=m  TranslationThetaOffset=0  TranslationThetaOffsetUnits=deg  RotationMethod=None  RotationAngleUnits=deg  RotationStandardAxis=+Z  RotationAngle=0  RotationArbitraryAxis=[0 0 1]  FollAlignAxisA=+X  BaseAlignAxisA=+Y  FollAlignAxisB=+Y  BaseAlignAxisB=+Z  RotationMatrix=[1 0 0; 0 1 0; 0 0 1]  BlockFunction=simmechanics.library.frames_transforms.rigid_transform
  Peg center transform3 : sm_lib/Frames and Transforms/Rigid Transform  TranslationMethod=StandardAxis  TranslationLengthUnit=cm  TranslationStandardAxis=+Z  TranslationStandardOffset=C_L/2  TranslationCartesianOffset=[0 0 0]  TranslationROffset=0  TranslationROffsetUnits=m  TranslationZOffset=0  TranslationZOffsetUnits=m  TranslationThetaOffset=0  TranslationThetaOffsetUnits=deg  RotationMethod=None  RotationAngleUnits=deg  RotationStandardAxis=+Z  RotationAngle=0  RotationArbitraryAxis=[0 0 1]  FollAlignAxisA=+X  BaseAlignAxisA=+Y  FollAlignAxisB=+Y  BaseAlignAxisB=+Z  RotationMatrix=[1 0 0; 0 1 0; 0 0 1]  BlockFunction=simmechanics.library.frames_transforms.rigid_transform
  BF : PMIOPort  Port=1  Side=Left
  FF : PMIOPort  Port=2  Side=Right
  connections:
  Peg center transform2/LConn1 -- Base/RConn1 -- Peg center transform1/RConn1
  FF/RConn1 -- Peg center transform3/RConn1
  Peg/RConn1 -- Peg center transform3/LConn1 -- Peg center transform2/RConn1
  BF/RConn1 -- Peg center transform1/LConn1

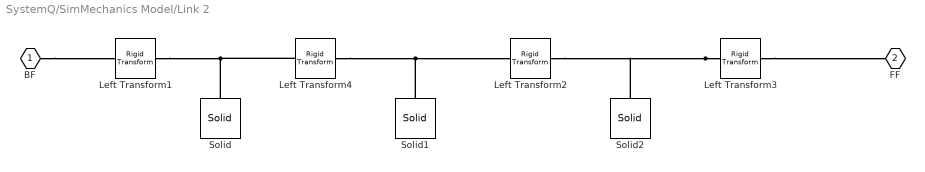
== system SystemQ/SimMechanics Model/Link 2 ==
  Left Transform1 : sm_lib/Frames and Transforms/Rigid Transform  TranslationMethod=StandardAxis  TranslationLengthUnit=cm  TranslationStandardAxis=+Z  TranslationStandardOffset=C_R/2  TranslationCartesianOffset=[0 0 0]  TranslationROffset=0  TranslationROffsetUnits=m  TranslationZOffset=0  TranslationZOffsetUnits=m  TranslationThetaOffset=0  TranslationThetaOffsetUnits=deg  RotationMethod=AlignedAxes  RotationAngleUnits=deg  RotationStandardAxis=+Y  RotationAngle=90  RotationArbitraryAxis=[0 0 1]  FollAlignAxisA=+Z  BaseAlignAxisA=+Z  FollAlignAxisB=+X  BaseAlignAxisB=+X  RotationMatrix=[1 0 0; 0 1 0; 0 0 1]  BlockFunction=simmechanics.library.frames_transforms.rigid_transform
  Left Transform2 : sm_lib/Frames and Transforms/Rigid Transform  TranslationMethod=Cartesian  TranslationLengthUnit=cm  TranslationStandardAxis=+Y  TranslationStandardOffset=-C_R/2  TranslationCartesianOffset="[C_R/2  0 C_L*0.5-7.5]"  TranslationROffset=0  TranslationROffsetUnits=m  TranslationZOffset=0  TranslationZOffsetUnits=m  TranslationThetaOffset=0  TranslationThetaOffsetUnits=deg  RotationMethod=AlignedAxes  RotationAngleUnits=deg  RotationStandardAxis=+Y  RotationAngle=90  RotationArbitraryAxis=[0 0 1]  FollAlignAxisA=+Z  BaseAlignAxisA=+X  FollAlignAxisB=+X  BaseAlignAxisB=+Z  RotationMatrix=[1 0 0; 0 1 0; 0 0 1]  BlockFunction=simmechanics.library.frames_transforms.rigid_transform
  Left Transform3 : sm_lib/Frames and Transforms/Rigid Transform  TranslationMethod=StandardAxis  TranslationLengthUnit=cm  TranslationStandardAxis=+Z  TranslationStandardOffset=C_R/2  TranslationCartesianOffset=[0 0 6*C_R]  TranslationROffset=0  TranslationROffsetUnits=m  TranslationZOffset=0  TranslationZOffsetUnits=m  TranslationThetaOffset=0  TranslationThetaOffsetUnits=deg  RotationMethod=None  RotationAngleUnits=deg  RotationStandardAxis=+Y  RotationAngle=90  RotationArbitraryAxis=[0 0 1]  FollAlignAxisA=+X  BaseAlignAxisA=+X  FollAlignAxisB=+Z  BaseAlignAxisB=+Z  RotationMatrix=[1 0 0; 0 1 0; 0 0 1]  BlockFunction=simmechanics.library.frames_transforms.rigid_transform
  Left Transform4 : sm_lib/Frames and Transforms/Rigid Transform  TranslationMethod=Cartesian  TranslationLengthUnit=cm  TranslationStandardAxis=+Y  TranslationStandardOffset=-C_R/2  TranslationCartesianOffset="[C_L*0.5-7.5  0 C_R/2]"  TranslationROffset=0  TranslationROffsetUnits=m  TranslationZOffset=0  TranslationZOffsetUnits=m  TranslationThetaOffset=0  TranslationThetaOffsetUnits=deg  RotationMethod=AlignedAxes  RotationAngleUnits=deg  RotationStandardAxis=+Y  RotationAngle=90  RotationArbitraryAxis=[0 0 1]  FollAlignAxisA=+Z  BaseAlignAxisA=+X  FollAlignAxisB=+X  BaseAlignAxisB=+Z  RotationMatrix=[1 0 0; 0 1 0; 0 0 1]  BlockFunction=simmechanics.library.frames_transforms.rigid_transform
  Solid : sm_lib/Body Elements/Solid  InertiaType=CalculateFromGeometry  Mass=1  MassUnits=kg  CenterOfMass=[0 0 0]  CenterOfMassUnits=m  MomentsOfInertia=[1 1 1]  MomentsOfInertiaUnits=kg*m^2  ProductsOfInertia=[0 0 0]  ProductsOfInertiaUnits=kg*m^2  DensityBased=on  Density=Ro  DensityUnits=kg/(m^3)  GraphicType=FromGeometry  MarkerShape=Sphere  MarkerSize=10  MarkerSizeUnits=m  GraphicVisPropType=SimpleVisualProperties  GraphicDiffuseColor=[0.0 0.0 0.0]  GraphicSpecularColor=[0.5 0.5 0.5 1.0]  GraphicAmbientColor=[0.15 0.15 0.15 1.0]  GraphicEmissiveColor=[0.0 0.0 0.0 1.0]  GraphicShininess=75  GraphicOpacity=1.0  GeometryShape=Cylinder  RectangleSize=[1 1]  RectangleSizeUnits=m  BrickDimensions=[1 1 1]  BrickDimensionUnits=m  CylinderRadius=5  CylinderRadiusUnits=cm  CylinderLength=C_R  CylinderLengthUnits=cm  SphereRadius=1  SphereRadiusUnits=m  EllipsoidRadii=[1 1 1]  EllipsoidRadiiUnits=m  ExtrusionCrossSection=[1 1; -1 1; -1 -1; 1 -1]  ExtrusionCrossSectionUnits=m  ExtrusionLength=1  ExtrusionLengthUnits=m  PolygonNumSides=3  PolygonOuterRadius=1  PolygonOuterRadiusUnits=m  ExtGeomFileType=STL  ExtGeomFileUnits=m  RevolutionCrossSection=[1 1; 1 -1; 2 -1; 2 1]  RevolutionCrossSectionUnits=m  RevolutionExtent=Full  RevolutionAngle=180  RevolutionAngleUnits=deg  BlockFunction=simmechanics.library.body_elements.solid
  Solid1 : sm_lib/Body Elements/Solid  InertiaType=CalculateFromGeometry  Mass=1  MassUnits=kg  CenterOfMass=[0 0 0]  CenterOfMassUnits=m  MomentsOfInertia=[1 1 1]  MomentsOfInertiaUnits=kg*m^2  ProductsOfInertia=[0 0 0]  ProductsOfInertiaUnits=kg*m^2  DensityBased=on  Density=Ro  DensityUnits=kg/(m^3)  GraphicType=FromGeometry  MarkerShape=Sphere  MarkerSize=10  MarkerSizeUnits=m  GraphicVisPropType=SimpleVisualProperties  GraphicDiffuseColor=[1.0 1.0 1.0]  GraphicSpecularColor=[0.5 0.5 0.5 1.0]  GraphicAmbientColor=[0.15 0.15 0.15 1.0]  GraphicEmissiveColor=[0.0 0.0 0.0 1.0]  GraphicShininess=75  GraphicOpacity=1.0  GeometryShape=Cylinder  RectangleSize=[1 1]  RectangleSizeUnits=m  BrickDimensions=[1 1 1]  BrickDimensionUnits=m  CylinderRadius=5  CylinderRadiusUnits=cm  CylinderLength=C_L  CylinderLengthUnits=cm  SphereRadius=1  SphereRadiusUnits=m  EllipsoidRadii=[1 1 1]  EllipsoidRadiiUnits=m  ExtrusionCrossSection=[1 1; -1 1; -1 -1; 1 -1]  ExtrusionCrossSectionUnits=m  ExtrusionLength=1  ExtrusionLengthUnits=m  PolygonNumSides=3  PolygonOuterRadius=1  PolygonOuterRadiusUnits=m  ExtGeomFileType=STL  ExtGeomFileUnits=m  RevolutionCrossSection=[1 1; 1 -1; 2 -1; 2 1]  RevolutionCrossSectionUnits=m  RevolutionExtent=Full  RevolutionAngle=180  RevolutionAngleUnits=deg  BlockFunction=simmechanics.library.body_elements.solid
  Solid2 : sm_lib/Body Elements/Solid  InertiaType=CalculateFromGeometry  Mass=1  MassUnits=kg  CenterOfMass=[0 0 0]  CenterOfMassUnits=m  MomentsOfInertia=[1 1 1]  MomentsOfInertiaUnits=kg*m^2  ProductsOfInertia=[0 0 0]  ProductsOfInertiaUnits=kg*m^2  DensityBased=on  Density=Ro  DensityUnits=kg/(m^3)  GraphicType=FromGeometry  MarkerShape=Sphere  MarkerSize=10  MarkerSizeUnits=m  GraphicVisPropType=SimpleVisualProperties  GraphicDiffuseColor=[0.0 0.0 0.0]  GraphicSpecularColor=[0.5 0.5 0.5 1.0]  GraphicAmbientColor=[0.15 0.15 0.15 1.0]  GraphicEmissiveColor=[0.0 0.0 0.0 1.0]  GraphicShininess=75  GraphicOpacity=1.0  GeometryShape=Cylinder  RectangleSize=[1 1]  RectangleSizeUnits=m  BrickDimensions=[1 1 1]  BrickDimensionUnits=m  CylinderRadius=5  CylinderRadiusUnits=cm  CylinderLength=C_R  CylinderLengthUnits=cm  SphereRadius=1  SphereRadiusUnits=m  EllipsoidRadii=[1 1 1]  EllipsoidRadiiUnits=m  ExtrusionCrossSection=[1 1; -1 1; -1 -1; 1 -1]  ExtrusionCrossSectionUnits=m  ExtrusionLength=1  ExtrusionLengthUnits=m  PolygonNumSides=3  PolygonOuterRadius=1  PolygonOuterRadiusUnits=m  ExtGeomFileType=STL  ExtGeomFileUnits=m  RevolutionCrossSection=[1 1; 1 -1; 2 -1; 2 1]  RevolutionCrossSectionUnits=m  RevolutionExtent=Full  RevolutionAngle=180  RevolutionAngleUnits=deg  BlockFunction=simmechanics.library.body_elements.solid
  BF : PMIOPort  Port=1  Side=Left
  FF : PMIOPort  Port=2  Side=Right
  connections:
  Left Transform3/LConn1 -- Solid2/RConn1 -- Left Transform2/RConn1
  Left Transform3/RConn1 -- FF/RConn1
  BF/RConn1 -- Left Transform1/LConn1
  Solid1/RConn1 -- Left Transform4/RConn1 -- Left Transform2/LConn1
  Solid/RConn1 -- Left Transform1/RConn1 -- Left Transform4/LConn1
